simulink model "RechargeAndPace"  (R2020a)
settings: Solver=FixedStepAuto  StartTime=0.0  StopTime=10.0  FixedStep=1e-3  RelTol=1e-3  EnableMultiTasking=on
undefined symbols (not defined in the file): D10, D11, D12, D2, D4, D5, D7, D8, D9, PTA0, PTA2, PTB23, PTB9, PTC3, PTC4, PTD0, PTD2, PTD3
libraries: frdmk64flib x11
settings Model: ExtModeTrigDuration=5  Creator=WinnieTrandinh  LastModifiedBy=WinnieTrandinh
settings OptimizationCC: EnhancedBackFolding=on  PassReuseOutputArgsAs=Individual arguments  ZeroExternalMemoryAtStartup=off  ZeroInternalMemoryAtStartup=off  MaxStackSize=64  OptimizeBlockOrder=speed  DifferentSizesBufferReuse=on  OptimizationCustomize=off  EfficientTunableParamExpr=on
settings DebuggingCC: ParameterTunabilityLossMsg=error
settings HardwareCC: ProdBitPerPointer=32  ProdBitPerSizeT=32  ProdBitPerPtrDiffT=32  ProdLargestAtomicInteger=Long  ProdLargestAtomicFloat=Double  ProdWordSize=32  ProdHWDeviceType=ARM Compatible->ARM Cortex
settings SFSimCC: MATLABDynamicMemAlloc=off
settings RTWCC: SystemTargetFile=ert.tlc  HardwareBoard=NXP FRDM-K64F  TemplateMakefile=ert_default_tmf  Toolchain=GNU Tools for ARM Embedded Processors
settings CodeAppCC: ForceParamTrailComments=on  IgnoreCustomStorageClasses=off  OperatorAnnotations=on  SimulinkDataObjDesc=on  SFDataObjDesc=on  InsertBlockDesc=on

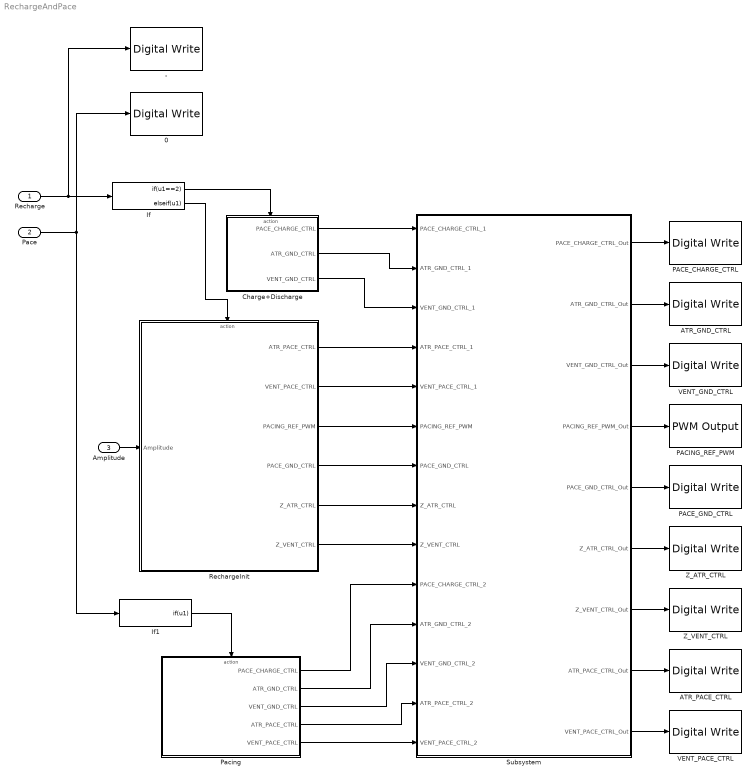
== system RechargeAndPace ==
  Recharge : Inport
  Pace : Inport  Port=2  OutDataTypeStr=boolean
  Amplitude : Inport  Port=3  Unit=V
  - : frdmk64flib/Digital Write  Whichpin=RED_LED
  0 : frdmk64flib/Digital Write  Whichpin=BLUE_LED
  ATR_GND_CTRL : frdmk64flib/Digital Write  Priority=2  Whichpin=PTD2 (D11)
  ATR_PACE_CTRL : frdmk64flib/Digital Write  Priority=4  Whichpin=PTA0 (D8)
  Charge+Discharge : Subsystem  TreatAsAtomicUnit=on
  If : If  IfExpression=u1==2  ElseIfExpressions=u1  ShowElse=off
  If1 : If  IfExpression=u1  ShowElse=off
  PACE_CHARGE_CTRL : frdmk64flib/Digital Write  Priority=1  Whichpin=PTB9 (D2)
  PACE_GND_CTRL : frdmk64flib/Digital Write  Priority=3  Whichpin=PTD0 (D10)
  PACING_REF_PWM : frdmk64flib/PWM Output  Priority=3  Whichpin=PTA2 (D5)  InitialFrequency=2000  InitialDutyCycle=20
  Pacing : Subsystem  TreatAsAtomicUnit=on
  RechargeInit : Subsystem  TreatAsAtomicUnit=on
  Subsystem : Subsystem
  VENT_GND_CTRL : frdmk64flib/Digital Write  Priority=2  Whichpin=PTD3 (D12)
  VENT_PACE_CTRL : frdmk64flib/Digital Write  Priority=4  Whichpin=PTC4 (D9)
  Z_ATR_CTRL : frdmk64flib/Digital Write  Priority=3  Whichpin=PTB23 (D4)
  Z_VENT_CTRL : frdmk64flib/Digital Write  Priority=3  Whichpin=PTC3 (D7)
  wires:
  Amplitude/1 -> RechargeInit/1(Amplitude)
  Recharge/1 -> -/1, If/1
  Pace/1 -> If1/1, 0/1
  If1/1 -> Pacing/Action
  If/2 -> RechargeInit/Action
  If/1 -> Charge+Discharge/Action
  Charge+Discharge/1(PACE_CHARGE_CTRL) -> Subsystem/1(PACE_CHARGE_CTRL_1)
  Charge+Discharge/2(ATR_GND_CTRL) -> Subsystem/2(ATR_GND_CTRL_1)
  Charge+Discharge/3(VENT_GND_CTRL) -> Subsystem/3(VENT_GND_CTRL_1)
  RechargeInit/2(VENT_PACE_CTRL) -> Subsystem/5(VENT_PACE_CTRL_1)
  RechargeInit/3(PACING_REF_PWM) -> Subsystem/6(PACING_REF_PWM)
  RechargeInit/4(PACE_GND_CTRL) -> Subsystem/7(PACE_GND_CTRL)
  RechargeInit/5(Z_ATR_CTRL) -> Subsystem/8(Z_ATR_CTRL)
  RechargeInit/6(Z_VENT_CTRL) -> Subsystem/9(Z_VENT_CTRL)
  Pacing/1(PACE_CHARGE_CTRL) -> Subsystem/10(PACE_CHARGE_CTRL_2)
  Pacing/2(ATR_GND_CTRL) -> Subsystem/11(ATR_GND_CTRL_2)
  Pacing/3(VENT_GND_CTRL) -> Subsystem/12(VENT_GND_CTRL_2)
  Pacing/4(ATR_PACE_CTRL) -> Subsystem/13(ATR_PACE_CTRL_2)
  Pacing/5(VENT_PACE_CTRL) -> Subsystem/14(VENT_PACE_CTRL_2)
  RechargeInit/1(ATR_PACE_CTRL) -> Subsystem/4(ATR_PACE_CTRL_1)
  Subsystem/1(PACE_CHARGE_CTRL_Out) -> PACE_CHARGE_CTRL/1
  Subsystem/2(ATR_GND_CTRL_Out) -> ATR_GND_CTRL/1
  Subsystem/3(VENT_GND_CTRL_Out) -> VENT_GND_CTRL/1
  Subsystem/4(PACING_REF_PWM_Out) -> PACING_REF_PWM/1
  Subsystem/5(PACE_GND_CTRL_Out) -> PACE_GND_CTRL/1
  Subsystem/6(Z_ATR_CTRL_Out) -> Z_ATR_CTRL/1
  Subsystem/7(Z_VENT_CTRL_Out) -> Z_VENT_CTRL/1
  Subsystem/8(ATR_PACE_CTRL_Out) -> ATR_PACE_CTRL/1
  Subsystem/9(VENT_PACE_CTRL_Out) -> VENT_PACE_CTRL/1

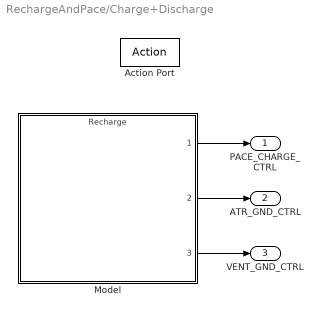
== system RechargeAndPace/Charge+Discharge ==
  Action Port : ActionPort  ActionPortLabel=if(u1==2)
  Model : ModelReference  ModelNameDialog=Recharge.slx  SimulationMode=Normal  ModelReferenceVersion=1.1
  PACE_CHARGE_CTRL : Outport
  ATR_GND_CTRL : Outport  Port=2
  VENT_GND_CTRL : Outport  Port=3
  wires:
  Model/2 -> ATR_GND_CTRL/1
  Model/1 -> PACE_CHARGE_CTRL/1
  Model/3 -> VENT_GND_CTRL/1

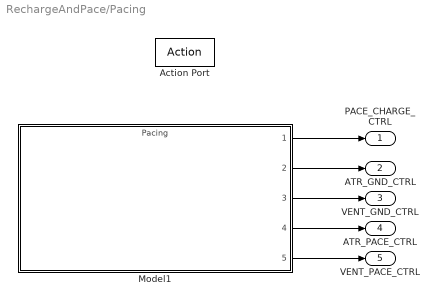
== system RechargeAndPace/Pacing ==
  Action Port : ActionPort  ActionPortLabel=if(u1)
  Model1 : ModelReference  ModelNameDialog=Pacing.slx  SimulationMode=Normal  ModelReferenceVersion=1.6
  PACE_CHARGE_CTRL : Outport
  ATR_GND_CTRL : Outport  Port=2
  VENT_GND_CTRL : Outport  Port=3
  ATR_PACE_CTRL : Outport  Port=4
  VENT_PACE_CTRL : Outport  Port=5
  wires:
  Model1/3 -> VENT_GND_CTRL/1
  Model1/2 -> ATR_GND_CTRL/1
  Model1/4 -> ATR_PACE_CTRL/1
  Model1/5 -> VENT_PACE_CTRL/1
  Model1/1 -> PACE_CHARGE_CTRL/1

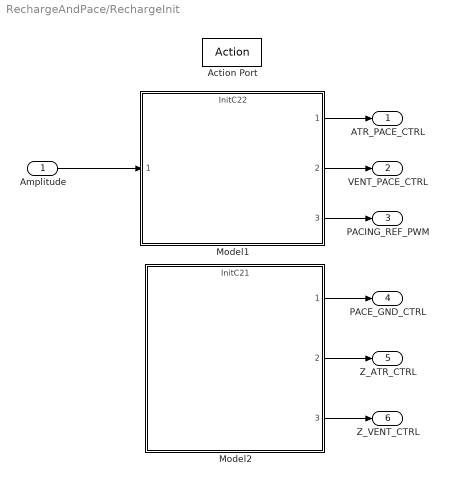
== system RechargeAndPace/RechargeInit ==
  Amplitude : Inport
  Action Port : ActionPort  ActionPortLabel=elseif(u1)
  Model1 : ModelReference  ModelNameDialog=InitC22.slx  SimulationMode=Normal  ModelReferenceVersion=1.15
  Model2 : ModelReference  ModelNameDialog=InitC21.slx  SimulationMode=Normal  ModelReferenceVersion=1.8
  ATR_PACE_CTRL : Outport
  VENT_PACE_CTRL : Outport  Port=2
  PACING_REF_PWM : Outport  Port=3
  PACE_GND_CTRL : Outport  Port=4
  Z_ATR_CTRL : Outport  Port=5
  Z_VENT_CTRL : Outport  Port=6
  wires:
  Amplitude/1 -> Model1/1
  Model1/1 -> ATR_PACE_CTRL/1
  Model1/2 -> VENT_PACE_CTRL/1
  Model1/3 -> PACING_REF_PWM/1
  Model2/1 -> PACE_GND_CTRL/1
  Model2/2 -> Z_ATR_CTRL/1
  Model2/3 -> Z_VENT_CTRL/1

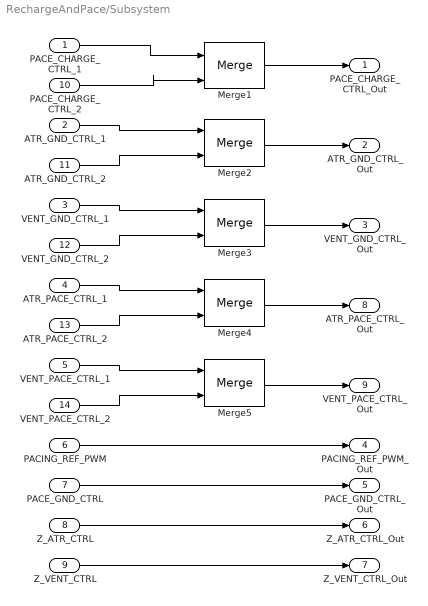
== system RechargeAndPace/Subsystem ==
  PACE_CHARGE_CTRL_1 : Inport
  ATR_GND_CTRL_1 : Inport  Port=2
  VENT_GND_CTRL_1 : Inport  Port=3
  ATR_PACE_CTRL_1 : Inport  Port=4
  VENT_PACE_CTRL_1 : Inport  Port=5
  PACING_REF_PWM : Inport  Port=6
  PACE_GND_CTRL : Inport  Port=7
  Z_ATR_CTRL : Inport  Port=8
  Z_VENT_CTRL : Inport  Port=9
  PACE_CHARGE_CTRL_2 : Inport  Port=10
  ATR_GND_CTRL_2 : Inport  Port=11
  VENT_GND_CTRL_2 : Inport  Port=12
  ATR_PACE_CTRL_2 : Inport  Port=13
  VENT_PACE_CTRL_2 : Inport  Port=14
  Merge{1..5} (5 alike) : Merge
  PACE_CHARGE_CTRL_Out : Outport
  ATR_GND_CTRL_Out : Outport  Port=2
  VENT_GND_CTRL_Out : Outport  Port=3
  PACING_REF_PWM_Out : Outport  Port=4
  PACE_GND_CTRL_Out : Outport  Port=5
  Z_ATR_CTRL_Out : Outport  Port=6
  Z_VENT_CTRL_Out : Outport  Port=7
  ATR_PACE_CTRL_Out : Outport  Port=8
  VENT_PACE_CTRL_Out : Outport  Port=9
  wires:
  PACE_CHARGE_CTRL_1/1 -> Merge1/1
  PACE_CHARGE_CTRL_2/1 -> Merge1/2
  Merge1/1 -> PACE_CHARGE_CTRL_Out/1
  ATR_GND_CTRL_1/1 -> Merge2/1
  ATR_GND_CTRL_2/1 -> Merge2/2
  Merge2/1 -> ATR_GND_CTRL_Out/1
  Merge3/1 -> VENT_GND_CTRL_Out/1
  VENT_GND_CTRL_2/1 -> Merge3/2
  VENT_GND_CTRL_1/1 -> Merge3/1
  Merge4/1 -> ATR_PACE_CTRL_Out/1
  ATR_PACE_CTRL_2/1 -> Merge4/2
  ATR_PACE_CTRL_1/1 -> Merge4/1
  Merge5/1 -> VENT_PACE_CTRL_Out/1
  VENT_PACE_CTRL_2/1 -> Merge5/2
  VENT_PACE_CTRL_1/1 -> Merge5/1
  PACING_REF_PWM/1 -> PACING_REF_PWM_Out/1
  PACE_GND_CTRL/1 -> PACE_GND_CTRL_Out/1
  Z_ATR_CTRL/1 -> Z_ATR_CTRL_Out/1
  Z_VENT_CTRL/1 -> Z_VENT_CTRL_Out/1
